simulink model "thermostat"  (R2022a)
settings: Solver=VariableStepAuto  StartTime=0.0  StopTime=10.0  MaxStep=0.2  RelTol=1e-3
values from neighbouring files (symbols this model uses):
  Ki = 0.05    [main.m]
  Kp = 0.50    (= 0.5)    [main.m]
  Ts = 0.15    [main.m]
settings Model: Creator=cc  LastModifiedBy=cc

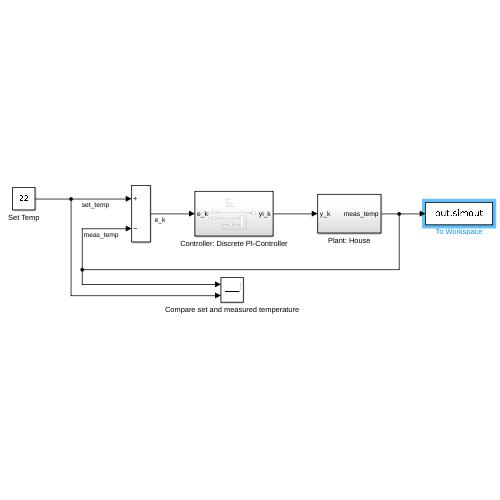
[thumbnail: Simulink's stored preview of the top-level diagram]
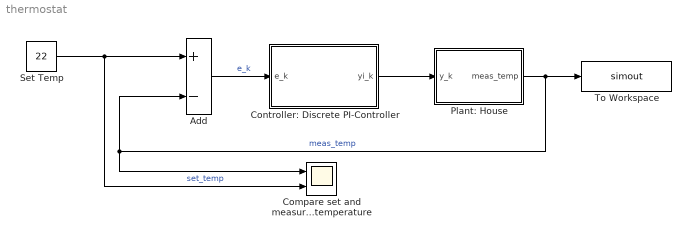
== system thermostat ==
  Add : Sum  Inputs=+-
  Compare set and measured temperature : Scope  NumInputPorts=2
  Controller: Discrete PI-Controller : Subsystem
  Plant: House : Subsystem
  Set Temp : Constant  Value=22
  To Workspace : ToWorkspace  VariableName=simout  SaveFormat=Timeseries  SampleTime=-1
  wires:
  Set Temp/1 -> Compare set and measured temperature/2, Add/1  "set_temp"
  Plant: House/1(meas_temp) -> To Workspace/1, Add/2, Compare set and measured temperature/1  "meas_temp"
  Add/1 -> Controller: Discrete PI-Controller/1(e_k)  "e_k"
  Controller: Discrete PI-Controller/1(yi_k) -> Plant: House/1(y_k)

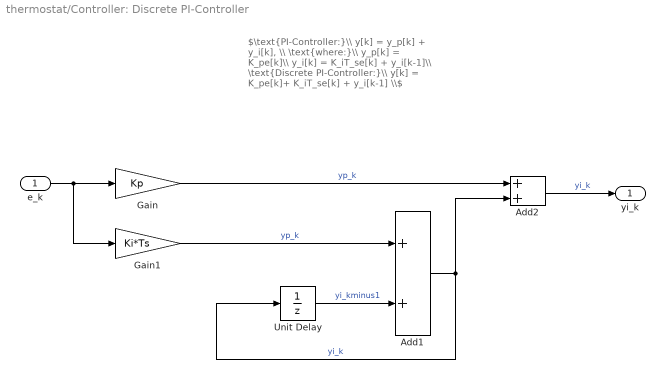
== system thermostat/Controller: Discrete PI-Controller ==
  note: $\text{PI-Controller:}\\ y[k] = y_p[k] + y_i[k], \\ \text{where:}\\ y_p[k] = K_pe[k]\\ y_i[k] = K_iT_se[k] + y_i[k-1]\\ \text{Discrete PI-Controller:}\\ y[k] = K_pe[k]+ K_iT_se[k] + y_i[k-1] \\$
  e_k : Inport
  Add1 : Sum
  Add2 : Sum
  Gain : Gain  Gain=Kp
  Gain1 : Gain  Gain=Ki*Ts
  Unit Delay : UnitDelay  SampleTime=Ts  HasFrameUpgradeWarning=on
  yi_k : Outport
  wires:
  Gain/1 -> Add2/1  "yp_k"
  Gain1/1 -> Add1/1  "yp_k"
  Unit Delay/1 -> Add1/2  "yi_kminus1"
  Add1/1 -> Add2/2, Unit Delay/1  "yi_k"
  e_k/1 -> Gain1/1, Gain/1
  Add2/1 -> yi_k/1  "yi_k"

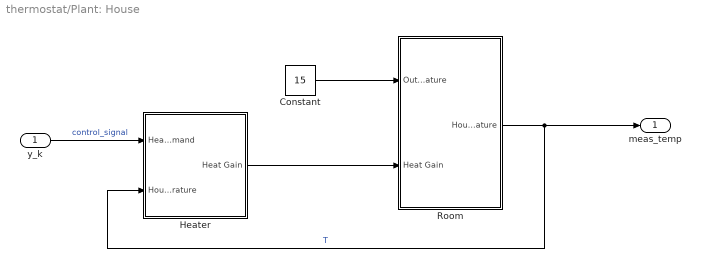
== system thermostat/Plant: House ==
  y_k : Inport
  Constant : Constant  Value=15
  Heater : Subsystem
  Room : Subsystem
  meas_temp : Outport  VectorParamsAs1DForOutWhenUnconnected=off
  wires:
  y_k/1 -> Heater/1(Heater Command)  "control_signal"
  Heater/1(Heat Gain) -> Room/2("Heat Gain ")
  Room/1(House Temperature) -> meas_temp/1, Heater/2(House Temperature)  "T"
  Constant/1 -> Room/1(Outside Temperature)

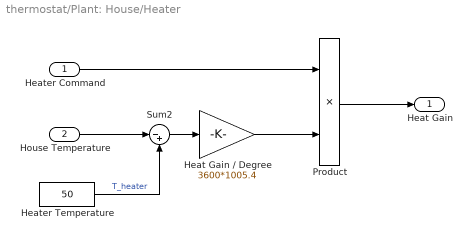
== system thermostat/Plant: House/Heater ==
  Heater Command : Inport
  House Temperature : Inport  Port=2
  Heat Gain / Degree : Gain  Gain=3600*1005.4
  Heater Temperature : Constant  Value=50
  Product : Product  RndMeth=Zero
  Sum2 : Sum  Inputs=|-+
  Heat Gain : Outport  Unit=joule/hour  VectorParamsAs1DForOutWhenUnconnected=off
  wires:
  Product/1 -> Heat Gain/1
  Heater Command/1 -> Product/1
  Heat Gain / Degree/1 -> Product/2
  Sum2/1 -> Heat Gain / Degree/1
  House Temperature/1 -> Sum2/1
  Heater Temperature/1 -> Sum2/2  "T_heater"

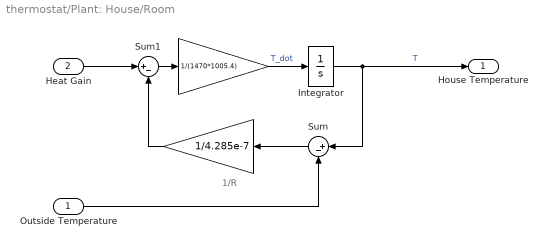
== system thermostat/Plant: House/Room ==
  note: 1/R
  Outside Temperature : Inport  Unit=°C
  "Heat Gain " : Inport  Port=2  Unit=joule/h
  " " : Gain  Gain=1/4.285e-7  SaturateOnIntegerOverflow=on  OutDataTypeStr=Inherit: Same as input  ParamDataTypeStr=Inherit: Same as input
  "  " : Gain  Gain=1/(1470*1005.4)  SaturateOnIntegerOverflow=on  OutDataTypeStr=Inherit: Same as input  ParamDataTypeStr=Inherit: Same as input
  Integrator : Integrator
  Sum : Sum  Inputs=|+-
  Sum1 : Sum  Inputs=|+-  InputSameDT=on  SaturateOnIntegerOverflow=on  OutDataTypeStr=Inherit: Same as first input
  House Temperature : Outport  Unit=°C  VectorParamsAs1DForOutWhenUnconnected=off
  wires:
  Outside Temperature/1 -> Sum/2
  Sum/1 -> " "/1
  " "/1 -> Sum1/2
  Integrator/1 -> House Temperature/1, Sum/1  "T"
  "  "/1 -> Integrator/1  "T_dot"
  Sum1/1 -> "  "/1
  "Heat Gain "/1 -> Sum1/1
